simulink model "Basic_Model"  (R2025b)
settings: Solver=VariableStepAuto  StartTime=0.0  StopTime=10.0  MaxStep=1e-3  RelTol=1e-3  AbsTol=1e-3  EnableMultiTasking=on
libraries: fl_lib x36, ee_lib x9, nesl_utility x3
settings SolverCC: AutoScaleAbsTol=off  AlgebraicLoopSolver=TrustRegion  MaxZcPerStep=1.0
settings DataIOCC: LimitDataPoints=on  MaxDataPoints=10000
settings OptimizationCC: ReuseModelBlockBuffer=off  LifeSpan=inf
settings DebuggingCC: UnconnectedInputMsg=warning  UnconnectedOutputMsg=warning  UnconnectedLineMsg=warning  AllowSymbolicDim=off  SFUnexpectedBacktrackingDiag=warning  SFNoUnconditionalDefaultTransitionDiag=warning  SFExecutionAtInitializationDiag=none  ArithmeticOperatorsInVariantConditions=warning
settings ModelReferenceCC: EnableRefExpFcnMdlSchedulingChecks=on
settings SFSimCC: SimUseLocalCustomCode=off  CustomCodeUndefinedFunction=UseInterfaceOnly
settings RTWCC: RTWUseLocalCustomCode=off  GPUComputeCapability=3.5  DLArmComputeVersion=19.05
settings CodeAppCC: StateflowObjectComments=on
settings GRTTargetCC: TargetLangStandard=C89/C90 (ANSI)
settings ConfigComp: CovMetricSettings=dw  CovSaveCumulativeToWorkspaceVar=on  CovSaveSingleToWorkspaceVar=on  CovExternalEMLEnable=off  CovSFcnEnable=off
settings SimscapeCC: SimscapeLogType=all  SimscapeLogSimulationStatistics=on  SimscapeLogDataHistory=10000.0

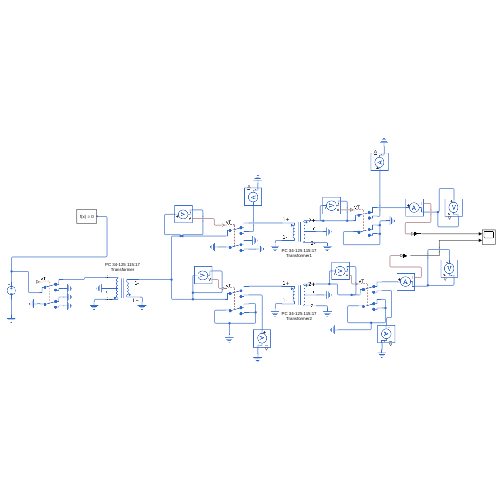
[thumbnail: Simulink's stored preview of the top-level diagram]
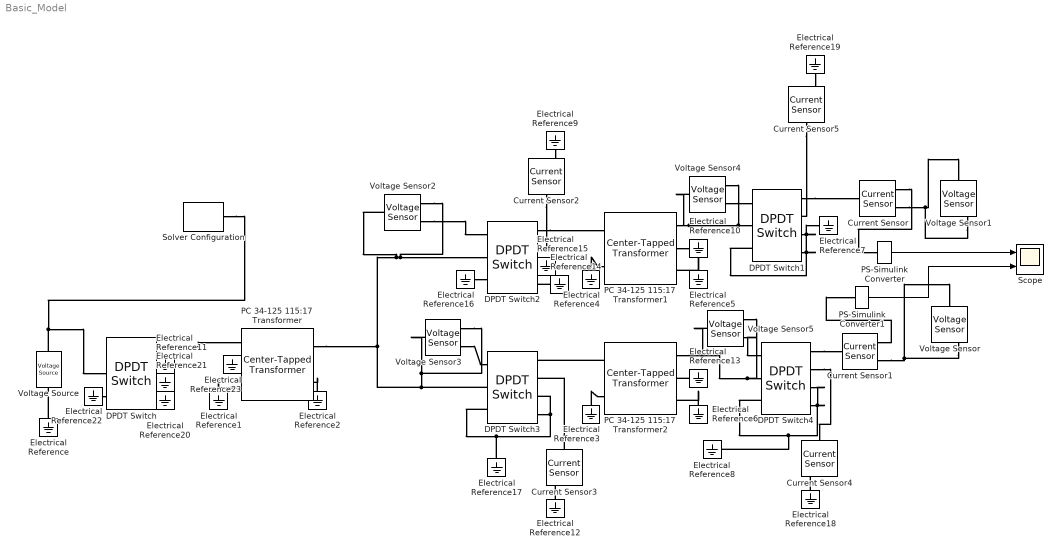
== system Basic_Model ==
  Current Sensor{,1..5} (6 alike) : fl_lib/Electrical/Electrical Sensors/Current Sensor
  DPDT Switch{,1..4} (5 alike) : ee_lib/Switches & Breakers/DPDT Switch  R_closed=0.01 Ohm  G_open=1e-6 S  Threshold=3.75 V  Width=0 V  model_dynamics=0  t_on=1e-3 s  t_off=1e-3 s  initial_vT=0 V
      settings: InternalSimscapePortConfiguration="{\"Bottom\":[],\"Left\":[{\"id\":\"vT\",\"label\":\"vT\",\"type\":\"input\"},{\"id\":\"p1\",\"label\":\"\",\"type\":\"foundation.electrical.electrical\"},{\"id\":\"p2\",\"label\":\"\",\"type\":\"foundation.electrical.electrical\"}],\"Right\":[{\"id\":\"n11\",\"label\":\"\",\"type\":\"foundation.electrical.electrical\"},{\"id\":\"n12\",\"label\":\"\",\"type\":\"foundation.electrical.electrical\"},{\"id\":\"n21\",\"label\":\"\",\"type\":\"foundation.electrical.electrical\"},{\"id\":\"n22\",\"label\":\"\",\"type\":\"foundation.electrical.electrical\"}],\"Top\":[]}"
  Electrical Reference{,1..23} (24 alike) : fl_lib/Electrical/Electrical Elements/Electrical Reference
  PC 34-125 115:17 Transformer : ee_lib/Passive/Transformers/Center-Tapped Transformer  modeling_option=ee.enum.transformer_option.ideal  n=3.3823529412  T=0.5  Rw1=0.01 Ohm  L1=0.0001 H  Rw2=0.01 Ohm  L2=0.0001 H  Rm=100 Ohm  Lm=0.04 H  i1_specify=off  i1_priority=None  i1=0 A  i1_nominal_specify=off  i1_nominal_value=1  i1_nominal_unit=A  i2p_specify=off  i2p_priority=None  i2p=0 A  i2p_nominal_specify=off  i2p_nominal_value=1  i2p_nominal_unit=A  i2n_specify=off  i2n_priority=None  i2n=0 A  i2n_nominal_specify=off  i2n_nominal_value=1  i2n_nominal_unit=A
      settings: InternalSimscapePortConfiguration="{\"Bottom\":[],\"Left\":[{\"id\":\"p1\",\"label\":\"1+\",\"type\":\"foundation.electrical.electrical\"},{\"id\":\"n1\",\"label\":\"1-\",\"type\":\"foundation.electrical.electrical\"}],\"Right\":[{\"id\":\"p2\",\"label\":\"2+\",\"type\":\"foundation.electrical.electrical\"},{\"id\":\"c\",\"label\":\"c\",\"type\":\"foundation.electrical.electrical\"},{\"id\":\"n2\",\"label\":\"2-\",\"type\":\"foundation.electrical.electrical\"}],\"Top\":[]}"
  PC 34-125 115:17 Transformer1 : ee_lib/Passive/Transformers/Center-Tapped Transformer  modeling_option=ee.enum.transformer_option.ideal  n=3.3823529412  T=0.5  Rw1=0.01 Ohm  L1=0.0001 H  Rw2=0.01 Ohm  L2=0.0001 H  Rm=100 Ohm  Lm=0.04 H  i1_specify=off  i1_priority=None  i1=0 A  i1_nominal_specify=off  i1_nominal_value=1  i1_nominal_unit=A  i2p_specify=off  i2p_priority=None  i2p=0 A  i2p_nominal_specify=off  i2p_nominal_value=1  i2p_nominal_unit=A  i2n_specify=off  i2n_priority=None  i2n=0 A  i2n_nominal_specify=off  i2n_nominal_value=1  i2n_nominal_unit=A
      settings: InternalSimscapePortConfiguration="{\"Bottom\":[],\"Left\":[{\"id\":\"p1\",\"label\":\"1+\",\"type\":\"foundation.electrical.electrical\"},{\"id\":\"n1\",\"label\":\"1-\",\"type\":\"foundation.electrical.electrical\"}],\"Right\":[{\"id\":\"p2\",\"label\":\"2+\",\"type\":\"foundation.electrical.electrical\"},{\"id\":\"c\",\"label\":\"c\",\"type\":\"foundation.electrical.electrical\"},{\"id\":\"n2\",\"label\":\"2-\",\"type\":\"foundation.electrical.electrical\"}],\"Top\":[]}"
  PC 34-125 115:17 Transformer2 : ee_lib/Passive/Transformers/Center-Tapped Transformer  modeling_option=ee.enum.transformer_option.ideal  n=3.3823529412  T=0.5  Rw1=0.01 Ohm  L1=0.0001 H  Rw2=0.01 Ohm  L2=0.0001 H  Rm=100 Ohm  Lm=0.04 H  i1_specify=off  i1_priority=None  i1=0 A  i1_nominal_specify=off  i1_nominal_value=1  i1_nominal_unit=A  i2p_specify=off  i2p_priority=None  i2p=0 A  i2p_nominal_specify=off  i2p_nominal_value=1  i2p_nominal_unit=A  i2n_specify=off  i2n_priority=None  i2n=0 A  i2n_nominal_specify=off  i2n_nominal_value=1  i2n_nominal_unit=A
      settings: InternalSimscapePortConfiguration="{\"Bottom\":[],\"Left\":[{\"id\":\"p1\",\"label\":\"1+\",\"type\":\"foundation.electrical.electrical\"},{\"id\":\"n1\",\"label\":\"1-\",\"type\":\"foundation.electrical.electrical\"}],\"Right\":[{\"id\":\"p2\",\"label\":\"2+\",\"type\":\"foundation.electrical.electrical\"},{\"id\":\"c\",\"label\":\"c\",\"type\":\"foundation.electrical.electrical\"},{\"id\":\"n2\",\"label\":\"2-\",\"type\":\"foundation.electrical.electrical\"}],\"Top\":[]}"
  PS-Simulink Converter : nesl_utility/PS-Simulink Converter  PhysicalDomain=network_engine_domain  SubClassName=ps_output  LeftPortType=input  RightPortType=output  PseudoPeriodic=off  Frequencies=[]  VectorFormat=inherit  Unit=inherit  AffineConversion=off
  PS-Simulink Converter1 : nesl_utility/PS-Simulink Converter  PhysicalDomain=network_engine_domain  SubClassName=ps_output  LeftPortType=input  RightPortType=output  PseudoPeriodic=off  Frequencies=[]  VectorFormat=inherit  Unit=inherit  AffineConversion=off
  Scope : Scope  NumInputPorts=2
      settings: ActiveDisplayYMinimum=-1  ActiveDisplayYMaximum=1
  Solver Configuration : nesl_utility/Solver Configuration  PhysicalDomain=network_engine_domain  SubClassName=solver  LeftPortType=input  RightPortType=generic  Tones=[]  Harmonics=[]  SimulateNoise=off  Profile=off  UseLocalSampling=off  EnableSwitchedLinearOptims=on  FrequencyDomain=off  UseCCode=off  RelTol=0.001  AbsTol=0.001  MinStep=1e-09  ToWorkspace=off  RevertToSquareIcSolve=off  NumHomotopyIterations=100  PhasorMode=off  PhasorModeNumHarmonics=1  ConsistencySolver=NEWTON_XTOL_AFTER_FTOL  IndexReductionMethod=DerivativeReplacement  DoDC=off  ResidualTolerance=1e-09  ConsistencyTolSource=GLOBAL  ConsistencyAbsTol=0.001  ConsistencyRelTol=0.001  ConsistencyTolFactor=0.001  UseLocalSolver=off  LocalSolverChoice=NE_BACKWARD_EULER_ADVANCER  ResolveIndetEquations=on  FunctionEvalNumThread=1  LocalSolverSampleTime=0.001  DoFixedCost=off  MaxNonlinIter=3  MaxModeIter=2  ComputeImpulses=off  ImpulseIterations=2  LinearAlgebra=auto  LinearAlgebraNumThread=0  EquationFormulation=NE_TIME_EF  DelaysMemoryBudget=1024  AutomaticFiltering=on  FilteringTimeConstant=0.001  PartitionStorageMethod=AS_NEEDED  PartitionMemoryBudget=1024  PartitionMethod=ROBUST  MultibodyUseLocalSolver=off  MultibodyLocalSolverChoice=ODE1  MultibodyLocalSolverSampleTime=0.001
  Voltage Sensor{,1..5} (6 alike) : fl_lib/Electrical/Electrical Sensors/Voltage Sensor
  Voltage Source : ee_lib/Sources/Voltage Source  dc_voltage=0 V  ac_voltage=0 V  ac_shift=0 rad  ac_frequency=60 Hz  noise_mode=ee.enum.sources.noise.Disabled  PSD=0 V^2/Hz  sample_time=1e-3 s  repeatability=ee.enum.sources.repeatability.NotRepeatable  user_seed=0  auto_seed=3499211588  i_specify=off  i_priority=None  i=0 A  i_nominal_specify=off  i_nominal_value=1  i_nominal_unit=A  v_specify=off  v_priority=None  v=0 V  v_nominal_specify=off  v_nominal_value=1  v_nominal_unit=V
  wires:
  PS-Simulink Converter/1 -> Scope/1
  PS-Simulink Converter1/1 -> Scope/2
  connections:
  Voltage Source/LConn1 -- Solver Configuration/RConn1 -- DPDT Switch/LConn2
  DPDT Switch/RConn1 -- PC 34-125 115:17 Transformer/RConn3
  DPDT Switch2/RConn1 -- PC 34-125 115:17 Transformer1/LConn1
  Electrical Reference/LConn1 -- Voltage Source/RConn1
  Electrical Reference1/LConn1 -- PC 34-125 115:17 Transformer/RConn1
  Electrical Reference2/LConn1 -- PC 34-125 115:17 Transformer/LConn1
  Electrical Reference4/LConn1 -- PC 34-125 115:17 Transformer1/LConn2
  Electrical Reference3/LConn1 -- PC 34-125 115:17 Transformer2/LConn2
  Electrical Reference5/LConn1 -- PC 34-125 115:17 Transformer1/RConn3
  Electrical Reference6/LConn1 -- PC 34-125 115:17 Transformer2/RConn3
  PC 34-125 115:17 Transformer/LConn2 -- Voltage Sensor3/RConn2 -- Voltage Sensor3/LConn1 -- DPDT Switch3/LConn2 -- Voltage Sensor2/LConn1 -- Voltage Sensor2/RConn2 -- DPDT Switch2/LConn2
  PC 34-125 115:17 Transformer2/LConn1 -- DPDT Switch3/RConn1
  PC 34-125 115:17 Transformer1/RConn1 -- Voltage Sensor4/LConn1 -- DPDT Switch1/LConn2 -- Voltage Sensor4/RConn2
  PC 34-125 115:17 Transformer2/RConn1 -- Voltage Sensor5/LConn1 -- Voltage Sensor5/RConn2 -- DPDT Switch4/LConn2
  DPDT Switch1/RConn1 -- Current Sensor/LConn1
  DPDT Switch4/RConn1 -- Current Sensor1/LConn1
  Current Sensor1/RConn2 -- Voltage Sensor/RConn2 -- Voltage Sensor/LConn1
  Current Sensor/RConn2 -- Voltage Sensor1/RConn2 -- Voltage Sensor1/LConn1
  DPDT Switch1/RConn3 -- DPDT Switch1/LConn3 -- DPDT Switch1/RConn4 -- Electrical Reference7/LConn1
  Electrical Reference8/LConn1 -- DPDT Switch4/RConn3 -- DPDT Switch4/RConn4 -- DPDT Switch4/LConn3
  Current Sensor3/LConn1 -- DPDT Switch3/RConn2
  Electrical Reference11/LConn1 -- DPDT Switch/RConn2
  Current Sensor/RConn1 -- PS-Simulink Converter/LConn1
  Current Sensor1/RConn1 -- PS-Simulink Converter1/LConn1
  Electrical Reference9/LConn1 -- Current Sensor2/RConn2
  Current Sensor2/LConn1 -- DPDT Switch2/RConn2
  Voltage Sensor2/RConn1 -- DPDT Switch2/LConn1
  Voltage Sensor3/RConn1 -- DPDT Switch3/LConn1
  Electrical Reference12/LConn1 -- Current Sensor3/RConn2
  Voltage Sensor4/RConn1 -- DPDT Switch1/LConn1
  Voltage Sensor5/RConn1 -- DPDT Switch4/LConn1
  PC 34-125 115:17 Transformer1/RConn2 -- Electrical Reference10/LConn1
  Electrical Reference13/LConn1 -- PC 34-125 115:17 Transformer2/RConn2
  Electrical Reference14/LConn1 -- DPDT Switch2/RConn4
  Electrical Reference15/LConn1 -- DPDT Switch2/RConn3
  Electrical Reference16/LConn1 -- DPDT Switch2/LConn3
  DPDT Switch3/RConn4 -- Electrical Reference17/LConn1 -- DPDT Switch3/LConn3 -- DPDT Switch3/RConn3
  Electrical Reference20/LConn1 -- DPDT Switch/RConn4
  Electrical Reference21/LConn1 -- DPDT Switch/RConn3
  Electrical Reference22/LConn1 -- DPDT Switch/LConn3
  Electrical Reference23/LConn1 -- PC 34-125 115:17 Transformer/RConn2
  Electrical Reference18/LConn1 -- Current Sensor4/RConn2
  DPDT Switch4/RConn2 -- Current Sensor4/LConn1
  Electrical Reference19/LConn1 -- Current Sensor5/RConn2
  Current Sensor5/LConn1 -- DPDT Switch1/RConn2
